simulink model "motor_model"  (R2022b)
settings: Solver=VariableStepAuto  StartTime=0.0  StopTime=10.0  RelTol=1e-3
settings Model: Creator=Y  LastModifiedBy=Y

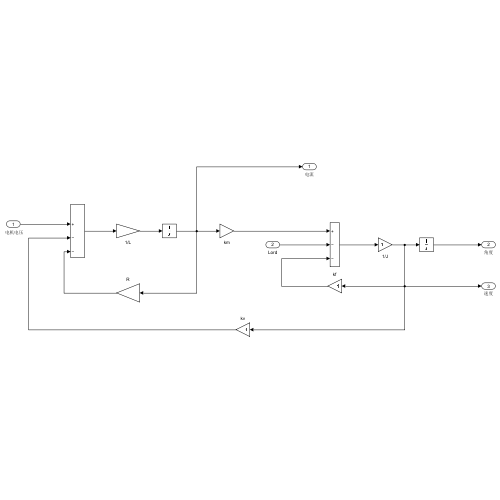
[thumbnail: Simulink's stored preview of the top-level diagram]
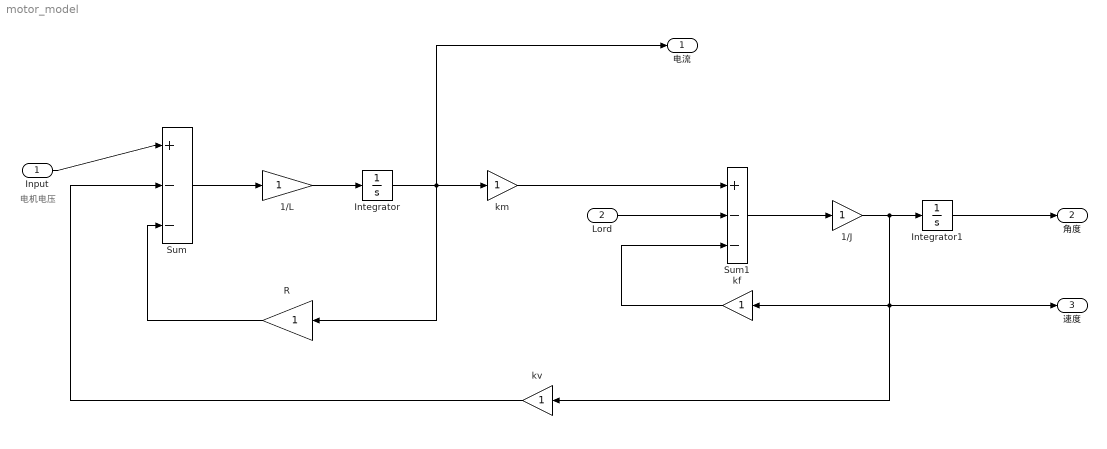
== system motor_model ==
  note: 电机电压
  Input : Inport
  Lord : Inport  Port=2
  1/J : Gain
  1/L : Gain
  Integrator : Integrator
  Integrator1 : Integrator
  R : Gain
  Sum : Sum  Inputs=|+--
  Sum1 : Sum  Inputs=+--
  kf : Gain
  km : Gain
  kv : Gain
  电流 : Outport
  角度 : Outport  Port=2
  速度 : Outport  Port=3
  wires:
  Input/1 -> Sum/1
  Sum/1 -> 1/L/1
  1/L/1 -> Integrator/1
  R/1 -> Sum/3
  Integrator/1 -> 电流/1, R/1, km/1
  km/1 -> Sum1/1
  Lord/1 -> Sum1/2
  Sum1/1 -> 1/J/1
  1/J/1 -> kv/1, 速度/1, kf/1, Integrator1/1
  Integrator1/1 -> 角度/1
  kf/1 -> Sum1/3
  kv/1 -> Sum/2
